simulink model "untitled"  (R2025b)
settings: Solver=VariableStepAuto  StartTime=0.0  StopTime=T_sim  RelTol=1e-3
values from neighbouring files (symbols this model uses):
  C1 = 1    [untitled1.m]
  C2 = 1    [untitled1.m]
  h1_ini = 0.7    [untitled1.m]
  h1_ref = 1    [untitled1.m]
  h2_ini = 0.6    [untitled1.m]
  h2_ref = 1.2    [untitled1.m]
  k = 0.05    [untitled1.m]
  u1_ref = k*sqrt(h2_ref)    [untitled1.m]
  u2_ref = u1_ref    [untitled1.m]
libraries: cstblocks x1
settings Model: Creator=leonardo  LastModifiedBy=leonardo

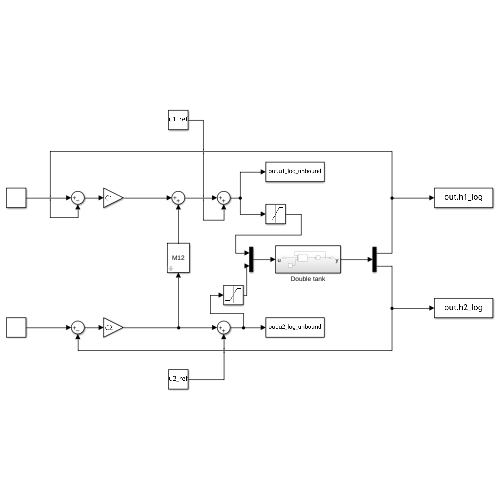
[thumbnail: Simulink's stored preview of the top-level diagram]
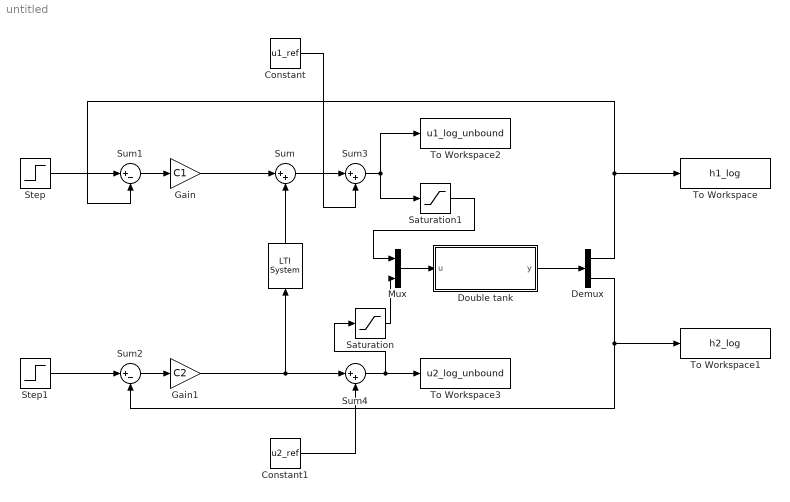
== system untitled ==
  " " : cstblocks/LTI System  sys=M12  IC=[]  PadeOrder=0
  Constant : Constant  Value=u1_ref
  Constant1 : Constant  Value=u2_ref
  Demux : Demux  Outputs=2
  Double tank : Subsystem
  Gain : Gain  Gain=C1
  Gain1 : Gain  Gain=C2
  Mux : Mux  Inputs=2
  Saturation : Saturate
  Saturation1 : Saturate
  Step : Step  Before=h1_ini  After=h1_ref  SampleTime=0
  Step1 : Step  Before=h2_ini  After=h2_ref  SampleTime=0
  Sum : Sum  Inputs=|++
  Sum1 : Sum  Inputs=|+-
  Sum2 : Sum  Inputs=|+-
  Sum3 : Sum  Inputs=|++
  Sum4 : Sum  Inputs=|++
  To Workspace : ToWorkspace  VariableName=h1_log  SaveFormat=Timeseries  SampleTime=-1
  To Workspace1 : ToWorkspace  VariableName=h2_log  SaveFormat=Timeseries  SampleTime=-1
  To Workspace2 : ToWorkspace  VariableName=u1_log_unbound  SaveFormat=Timeseries  SampleTime=-1
  To Workspace3 : ToWorkspace  VariableName=u2_log_unbound  SaveFormat=Timeseries  SampleTime=-1
  wires:
  Gain/1 -> Sum/1
  " "/1 -> Sum/2
  Mux/1 -> Double tank/1(u)
  Double tank/1(y) -> Demux/1
  Step/1 -> Sum1/1
  Sum1/1 -> Gain/1
  Sum2/1 -> Gain1/1
  Step1/1 -> Sum2/1
  Demux/1 -> Sum1/2, To Workspace/1
  Demux/2 -> To Workspace1/1, Sum2/2
  Gain1/1 -> Sum4/1, " "/1
  Sum/1 -> Sum3/1
  Constant/1 -> Sum3/2
  Constant1/1 -> Sum4/2
  Sum4/1 -> Saturation/1, To Workspace3/1
  Sum3/1 -> Saturation1/1, To Workspace2/1
  Saturation/1 -> Mux/2
  Saturation1/1 -> Mux/1

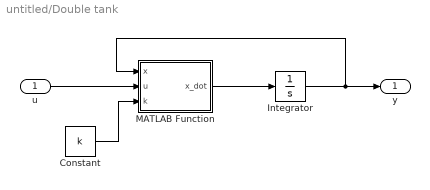
== system untitled/Double tank ==
  u : Inport
  Constant : Constant  Value=k
  Integrator : Integrator  InitialCondition=[h1_ini;h2_ini]
  MATLAB Function : MATLAB Function  TreatAsAtomicUnit=on
  y : Outport
  wires:
  u/1 -> MATLAB Function/2(u)
  MATLAB Function/1(x_dot) -> Integrator/1
  Integrator/1 -> MATLAB Function/1(x), y/1
  Constant/1 -> MATLAB Function/3(k)

== matlab function untitled/Double tank/MATLAB Function ==
  data: x_dot output; x input; u input; k input
function x_dot = double_tank(x, u, k)
x_dot = zeros(2, 1);

x_dot(1) = u(1) - u(2);
x_dot(2) = u(2) - k*sqrt(x(2));
